simulink model "poleplacement_2019b"  (R2019b)
settings: Solver=VariableStepAuto  StartTime=0.0  StopTime=10.0  RelTol=1e-3
values from neighbouring files (symbols this model uses):
  k = place(sysestc.A, sysestc.B, new_pole)    [PolePlacement.m]    (also in PolePlacement_Controller_script.m = place(A, B, new_pole); ppObs.m = place(A, B, new_pole))
  k2 = place(sysest.A, sysest.B, new_pole2)    [PolePlacement.m]    (also in PolePlacement_Controller_script.m; ppObs.m)
  K_eta = K_en(5)    [PolePlacement_Controller_script.m]    (also in ppObs.m)
  K_x = K_en(1:4)    [PolePlacement_Controller_script.m]    (also in ppObs.m)
  Kr = 1/Kdc(1)    [PolePlacement.m]    (also in PolePlacement_Controller_script.m; ppObs.m = 1/Kdc)
  Kr2 = 1/Kdc2    [PolePlacement.m]    (also in PolePlacement_Controller_script.m; ppObs.m)
  L = place(sysestc.A',sysestc.C', 10*new_pole)'    [PolePlacement.m]    (also in PolePlacement_Controller_script.m; ppObs.m = place(A',C', 10*new_pole)')
  L22 = place(sysest.A',sysest.C', new_pole2/0.99)'    [PolePlacement.m]    (also in PolePlacement_Controller_script.m; ppObs.m)
  sysest = load("sysest.mat").sysest    [PolePlacement.m]    (also in PolePlacement_Controller_script.m = load("sysest_matching.mat").sysest; ppObs.m)
  sysestc = d2c(sysest)    [PolePlacement.m]    (also in PolePlacement_Controller_script.m; ppObs.m)
undefined symbols (not defined in the file or in its folder): DiscIntNeverNeededParam, sigbuilder_block
libraries: simulink_extras x7, cstblocks x4, simulink x1
settings Model: Creator=jesuc  LastModifiedBy=AleFire
settings DebuggingCC: SFMachineParentedDataDiag=error

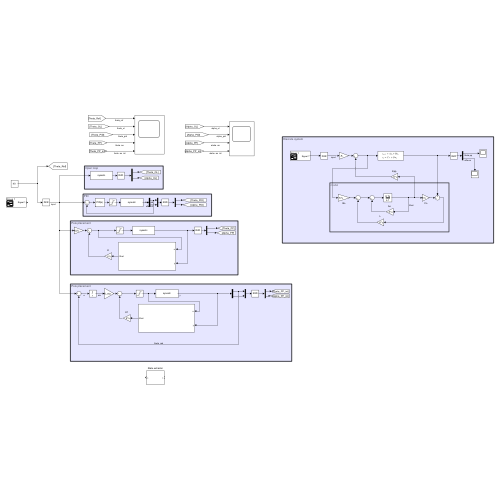
[thumbnail: Simulink's stored preview of the top-level diagram]
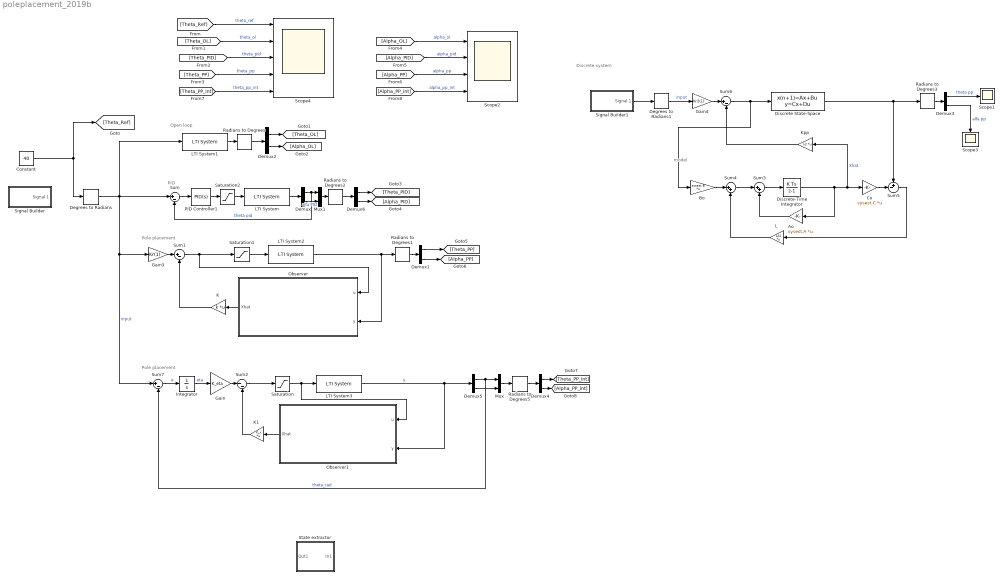
== system poleplacement_2019b ==
  note: Discrete system
  note: Pole placement
  note: PID
  note: Open loop
  note: model
  note: Pole placement
  Ao : Gain  Gain=sysest.A  Multiplication=Matrix(K*u)
  Bo : Gain  Gain=sysest.B  Multiplication=Matrix(K*u)
  Co : Gain  Gain=sysest.C  Multiplication=Matrix(K*u)
  Constant : Constant  Value=40
  Degrees to Radians : simulink_extras/Transformations/Degrees to Radians
  Degrees to Radians1 : simulink_extras/Transformations/Degrees to Radians
  Demux{,1..6} (7 alike) : Demux  Outputs=2
  Discrete State-Space : DiscreteStateSpace  A=sysest.A  B=sysest.B  C=sysest.C  D=sysest.D  SampleTime=0.002
  Discrete-Time Integrator : DiscreteIntegrator  SampleTime=0.002  ICPrevOutput=DiscIntNeverNeededParam  ICPrevScaledInput=DiscIntNeverNeededParam
  Gain : Gain  Gain=K_eta
  Gain3 : Gain  Gain=Kr(1)
  Gain4 : Gain  Gain=Kr2(1)
  Integrator : Integrator
  K : Gain  Gain=k  Multiplication=Matrix(K*u)
  K1 : Gain  Gain=K_x  Multiplication=Matrix(K*u)
  Kpp : Gain  Gain=k2  Multiplication=Matrix(K*u)
  L : Gain  Gain=L22  Multiplication=Matrix(K*u)
  LTI System{,1..3} (4 alike) : cstblocks/LTI System  sys=sysestc  IC=[]
  Mux : Mux  Inputs=2
  Mux1 : Mux  Inputs=2
  Observer : Subsystem
  Observer1 : Subsystem
  PID Controller1 : simulink/Continuous/PID Controller  Controller=PID  Form=Parallel  TimeDomain=Continuous-time  SampleTime=-1  IntegratorMethod=Forward Euler  FilterMethod=Forward Euler  ControllerParametersSource=internal  P=1  I=1  D=0  N=100  UseFilter=on  TunerSelectOption=Transfer Function Based (PID Tuner App)  InitialConditionSource=internal  InitialConditionForIntegrator=0  InitialConditionForFilter=0  DifferentiatorICPrevScaledInput=0  ExternalReset=none  TrackingMode=off  Kt=1  LimitOutput=off  UpperSaturationLimit=inf  LowerSaturationLimit=-inf  LinearizeAsGain=on  AntiWindupMode=none  Kb=1  POutMin=[]  POutMax=[]  IOutMin=[]  IOutMax=[]  DOutMin=[]  DOutMax=[]  NOutMin=[]  NOutMax=[]  SumOutMin=[]  SumOutMax=[]  SaturationOutMin=[]  SaturationOutMax=[]  PParamMin=[]  PParamMax=[]  IParamMin=[]  IParamMax=[]  DParamMin=[]  DParamMax=[]  NParamMin=[]  NParamMax=[]  KbParamMin=[]  KbParamMax=[]  KtParamMin=[]  KtParamMax=[]  KbOutMin=[]  KbOutMax=[]  KtOutMin=[]  KtOutMax=[]  IntegratorOutMin=[]  IntegratorOutMax=[]  FilterOutMin=[]  FilterOutMax=[]  SumI1OutMin=[]  SumI1OutMax=[]  SumI2OutMin=[]  SumI2OutMax=[]  SumI3OutMin=[]  SumI3OutMax=[]  SumI4OutMin=[]  SumI4OutMax=[]  SumDOutMin=[]  SumDOutMax=[]  DifferentiatorOutMin=[]  DifferentiatorOutMax=[]  FilterDiffOutCoefMin=[]  FilterDiffOutCoefMax=[]  ReciprocalOutMin=[]  ReciprocalOutMax=[]  SumDenOutMin=[]  SumDenOutMax=[]  SumNumOutMin=[]  SumNumOutMax=[]  DivideOutMin=[]  DivideOutMax=[]  IntegratorContinuousStateAttributes=''  IntegratorStateMustResolveToSignalObject=off  IntegratorRTWStateStorageClass=Auto  FilterContinuousStateAttributes=''  FilterStateMustResolveToSignalObject=off  FilterRTWStateStorageClass=Auto  ParallelPVariant=InternalParameters  IdealPVariant=Disabled  IVariant=InternalParameters  DVariant=InternalParameters  IntegratorVariant=Continuous  SatVariant=Disabled  AWVariant=Passthrough  PCopyVariant=Disabled  TRVariant=Disabled  FdbkBlocksVariant=Forward  IdealPFdbkVariant=Disabled  SatFdbkVariant=Disabled  DerivativeFilterVariant=ContFilter  NVariant=InternalParameters  NCopyVariant=Disabled  FilterICVariant=InternalICsFilter  IntegratorICVariant=InternalICs  ExternalResetVariant=Disabled  TRSumVariant=Passthrough  SumFdbkVariant=Disabled  SumVariant=Sum_PID
  Radians to Degrees{,1..3,5} (5 alike) : simulink_extras/Transformations/Radians to Degrees
  Saturation : Saturate  UpperLimit=4.5  LowerLimit=-4.5
  Saturation1 : Saturate  UpperLimit=4.5  LowerLimit=-4.5
  Saturation2 : Saturate  UpperLimit=4.5  LowerLimit=-4.5
  Scope1 : Scope
  Scope2 : Scope  NumInputPorts=4
  Scope3 : Scope
  Scope4 : Scope  NumInputPorts=5
  Signal Builder : Subsystem  Tag=STV Subsys  LoadFcn=sigbuilder_block('load');  StartFcn=sigbuilder_block('start');  StopFcn=sigbuilder_block('stop');  ClipboardFcn=sigbuilder_block('clipboard');  mask(Sigbuilder block){tuvar=[0:10]}
      mask help: Simulink:masks:SigbuilderBlock_MD
      mask init:
      | if ~strcmp(get_param(bdroot(gcbh),'SimulationStatus'),'stopped') tuvar = sigbuilder_block('maskInit'); end
      settings: CopyFcn=sigbuilder_block('copy');  DeleteFcn=sigbuilder_block('delete');  ModelCloseFcn=sigbuilder_block('modelClose');  PreSaveFcn=sigbuilder_block('preSave');  PauseFcn=sigbuilder_block('pause');  ContinueFcn=sigbuilder_block('continue');  NameChangeFcn=sigbuilder_block('namechange');  OpenFcn=sigbuilder_block('open',[437.6 199.2 550.4 400 ]);  CloseFcn=sigbuilder_block('close');
      mask Display: plot(0, 0, 100, 100,[2, 2, 32, 32, 2], [68, 8, 8, 68, 68],[32, 2], [38, 38], [32, 19, 2],[53, 60, 44], [32, 17, 17, 2],[16, 16, 31, 31]);txt = getActiveGroup(gcbh);text(2, 100, txt,'verticalAlignment', 'top');
  Signal Builder1 : Subsystem  Tag=STV Subsys  LoadFcn=sigbuilder_block('load');  StartFcn=sigbuilder_block('start');  StopFcn=sigbuilder_block('stop');  ClipboardFcn=sigbuilder_block('clipboard');  mask(Sigbuilder block){tuvar=[0:10]}
      mask help: Simulink:masks:SigbuilderBlock_MD
      mask init:
      | if ~strcmp(get_param(bdroot(gcbh),'SimulationStatus'),'stopped') tuvar = sigbuilder_block('maskInit'); end
      settings: CopyFcn=sigbuilder_block('copy');  DeleteFcn=sigbuilder_block('delete');  ModelCloseFcn=sigbuilder_block('modelClose');  PreSaveFcn=sigbuilder_block('preSave');  PauseFcn=sigbuilder_block('pause');  ContinueFcn=sigbuilder_block('continue');  NameChangeFcn=sigbuilder_block('namechange');  OpenFcn=sigbuilder_block('open',[437.6 199.2 550.4 400 ]);  CloseFcn=sigbuilder_block('close');
      mask Display: plot(0, 0, 100, 100,[2, 2, 32, 32, 2], [68, 8, 8, 68, 68],[32, 2], [38, 38], [32, 19, 2],[53, 60, 44], [32, 17, 17, 2],[16, 16, 31, 31]);txt = getActiveGroup(gcbh);text(2, 100, txt,'verticalAlignment', 'top');
  State extractor : Subsystem
  Sum{,1,6..7} (4 alike) : Sum  Inputs=|+-
  Sum2 : Sum  Inputs=|--
  Sum3 : Sum  Inputs=|++
  Sum4 : Sum  Inputs=|++
  Sum5 : Sum  Inputs=+-|
  wires:
  Degrees to Radians/1 -> Sum/1, Gain3/1, Sum7/1, LTI System1/1  "input"
  Sum/1 -> PID Controller1/1
  LTI System/1 -> Demux/1
  Demux/1 -> Mux1/1, Sum/2  "theta pid"
  K/1 -> Sum1/2
  Gain3/1 -> Sum1/1
  Demux/2 -> Mux1/2  "alfa PID"
  Sum1/1 -> Saturation1/1, Observer/1(u)
  Observer/1(Xhat) -> K/1
  LTI System1/1 -> Radians to Degrees/1
  Demux2/1 -> [Theta_OL]
  Demux2/2 -> [Alpha_OL]
  Demux3/1 -> Scope1/1  "theta pp"
  Kpp/1 -> Sum6/2
  Sum4/1 -> Sum3/1
  Sum3/1 -> Discrete-Time Integrator/1
  Bo/1 -> Sum4/1
  Co/1 -> Sum5/2
  Gain4/1 -> Sum6/1
  Ao/1 -> Sum3/2
  L/1 -> Sum4/2
  Discrete-Time Integrator/1 -> Ao/1, Kpp/1, Co/1  "Xhat"
  Discrete State-Space/1 -> Radians to Degrees3/1, Sum5/1
  Sum5/1 -> L/1
  Sum6/1 -> Discrete State-Space/1, Bo/1
  Degrees to Radians1/1 -> Gain4/1  "input"
  Demux3/2 -> Scope3/1  "alfa pp"
  Radians to Degrees3/1 -> Demux3/1
  Constant/1 -> Degrees to Radians/1, [Theta_Ref]
  Signal Builder1/1(Signal 1) -> Degrees to Radians1/1
  Radians to Degrees/1 -> Demux2/1
  [Theta_Ref] -> Scope4/1  "theta_ref"
  [Theta_OL] -> Scope4/2  "theta_ol"
  [Theta_PID] -> Scope4/3  "theta_pid"
  LTI System2/1 -> Radians to Degrees1/1, Observer/2(y)
  Radians to Degrees1/1 -> Demux1/1
  Demux1/1 -> [Theta_PP]
  Demux1/2 -> [Alpha_PP]
  [Theta_PP] -> Scope4/4  "theta_pp"
  [Alpha_OL] -> Scope2/1  "alpha_ol"
  [Alpha_PID] -> Scope2/2  "alpha_pid"
  [Alpha_PP] -> Scope2/3  "alpha_pp"
  Radians to Degrees5/1 -> Demux4/1
  LTI System3/1 -> Observer1/2(y), Demux5/1  "y"
  Demux4/2 -> [Alpha_PP_int]
  K1/1 -> Sum2/2
  Sum2/1 -> Saturation/1
  Demux4/1 -> [Theta_PP_int]
  Sum7/1 -> Integrator/1  "e"
  Gain/1 -> Sum2/1
  [Theta_PP_int] -> Scope4/5  "theta_pp_int"
  [Alpha_PP_int] -> Scope2/4  "alpha_pp_int"
  Demux5/1 -> Sum7/2, Mux/1  "theta_rad"
  Demux5/2 -> Mux/2
  Mux/1 -> Radians to Degrees5/1
  Demux6/1 -> [Theta_PID]
  Radians to Degrees2/1 -> Demux6/1
  Demux6/2 -> [Alpha_PID]
  Mux1/1 -> Radians to Degrees2/1
  Saturation/1 -> Observer1/1(u), LTI System3/1
  Saturation1/1 -> LTI System2/1
  PID Controller1/1 -> Saturation2/1
  Saturation2/1 -> LTI System/1
  Integrator/1 -> Gain/1  "eta"
  Observer1/1(Xhat) -> K1/1

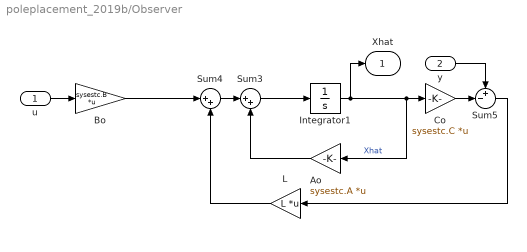
== system poleplacement_2019b/Observer ==
  u : Inport
  y : Inport  Port=2
  Ao : Gain  Gain=sysestc.A  Multiplication=Matrix(K*u)
  Bo : Gain  Gain=sysestc.B  Multiplication=Matrix(K*u)
  Co : Gain  Gain=sysestc.C  Multiplication=Matrix(K*u)
  Integrator1 : Integrator
  L : Gain  Gain=L  Multiplication=Matrix(K*u)
  Sum3 : Sum  Inputs=|++
  Sum4 : Sum  Inputs=|++
  Sum5 : Sum  Inputs=+-|
  Xhat : Outport
  wires:
  Sum5/1 -> L/1
  Sum4/1 -> Sum3/1
  u/1 -> Bo/1
  Sum3/1 -> Integrator1/1
  Integrator1/1 -> Ao/1, Co/1, Xhat/1  "Xhat"
  Ao/1 -> Sum3/2
  L/1 -> Sum4/2
  Co/1 -> Sum5/2
  Bo/1 -> Sum4/1
  y/1 -> Sum5/1

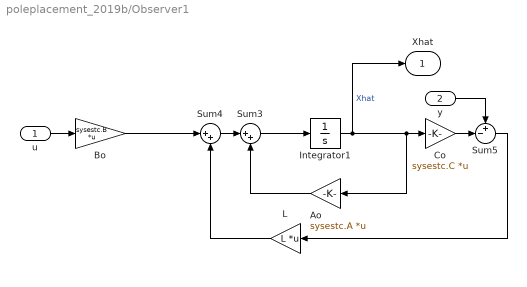
== system poleplacement_2019b/Observer1 ==
  u : Inport
  y : Inport  Port=2
  Ao : Gain  Gain=sysestc.A  Multiplication=Matrix(K*u)
  Bo : Gain  Gain=sysestc.B  Multiplication=Matrix(K*u)
  Co : Gain  Gain=sysestc.C  Multiplication=Matrix(K*u)
  Integrator1 : Integrator
  L : Gain  Gain=L  Multiplication=Matrix(K*u)
  Sum3 : Sum  Inputs=|++
  Sum4 : Sum  Inputs=|++
  Sum5 : Sum  Inputs=+-|
  Xhat : Outport
  wires:
  Sum5/1 -> L/1
  Sum4/1 -> Sum3/1
  u/1 -> Bo/1
  Sum3/1 -> Integrator1/1
  Integrator1/1 -> Xhat/1, Ao/1, Co/1  "Xhat"
  Ao/1 -> Sum3/2
  L/1 -> Sum4/2
  Co/1 -> Sum5/2
  Bo/1 -> Sum4/1
  y/1 -> Sum5/1

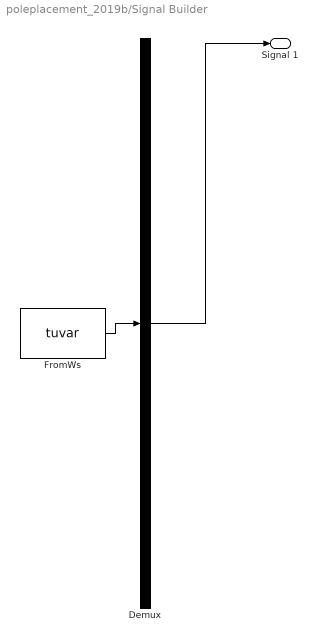
== system poleplacement_2019b/Signal Builder ==
  Demux : Demux  Tag=STV Demux  Outputs=1
      settings: DisplayOption=none
  FromWs : FromWorkspace  Tag=STV FromWs  VariableName=tuvar
      SigBuilderData=|
      | common.afterFinalStr = 'Extrapolate'
      | common.sampleTime = 0
      | dataSet.timeRange = [0 10]
      | dataSet.name = 'Group 1'
      | sbobj.Groups.Name = 'Group 1'
      | sbobj.Groups.Signals.Name = 'Signal 1'
      | sbobj.Groups.Signals.XData = [0 1 1 3 3 5 5 7 7 8.5 8.5 10]
      | sbobj.Groups.Signals.YData = [0.005 0.005 40 40 15 15 -30 -30 0 0 23 23]
  Signal 1 : Outport  Tag=STV Outport
  wires:
  Demux/1 -> Signal 1/1
  FromWs/1 -> Demux/1

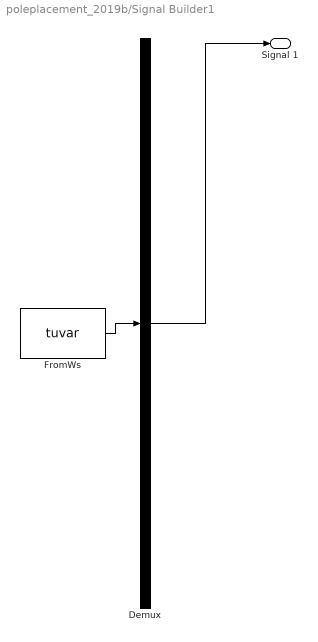
== system poleplacement_2019b/Signal Builder1 ==
  Demux : Demux  Tag=STV Demux  Outputs=1
      settings: DisplayOption=none
  FromWs : FromWorkspace  Tag=STV FromWs  VariableName=tuvar
      SigBuilderData=|
      | common.afterFinalStr = 'Extrapolate'
      | common.sampleTime = 0
      | dataSet.timeRange = [0 10]
      | dataSet.name = 'Group 1'
      | sbobj.Groups.Name = 'Group 1'
      | sbobj.Groups.Signals.Name = 'Signal 1'
      | sbobj.Groups.Signals.XData = [0 1 1 3 3 5 5 7 7 8.5 8.5 10]
      | sbobj.Groups.Signals.YData = [0.005 0.005 40 40 15 15 -30 -30 0 0 23 23]
  Signal 1 : Outport  Tag=STV Outport
  wires:
  Demux/1 -> Signal 1/1
  FromWs/1 -> Demux/1

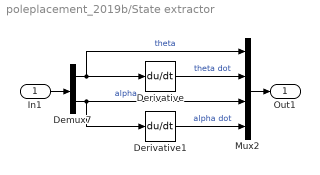
== system poleplacement_2019b/State extractor ==
  In1 : Inport
  Demux7 : Demux  Outputs=2
  Derivative : Derivative
  Derivative1 : Derivative
  Mux2 : Mux
  Out1 : Outport
  wires:
  In1/1 -> Demux7/1
  Derivative1/1 -> Mux2/4  "alpha dot"
  Derivative/1 -> Mux2/2  "theta dot"
  Demux7/1 -> Mux2/1, Derivative/1  "theta"
  Demux7/2 -> Derivative1/1, Mux2/3  "alpha"
  Mux2/1 -> Out1/1
